simulink model "pd_discreto"  (R2025b)
settings: Solver=VariableStepAuto  StartTime=0.0  StopTime=3  RelTol=1e-3
libraries: simulink x4
settings Model: Creator=rel  LastModifiedBy=rel

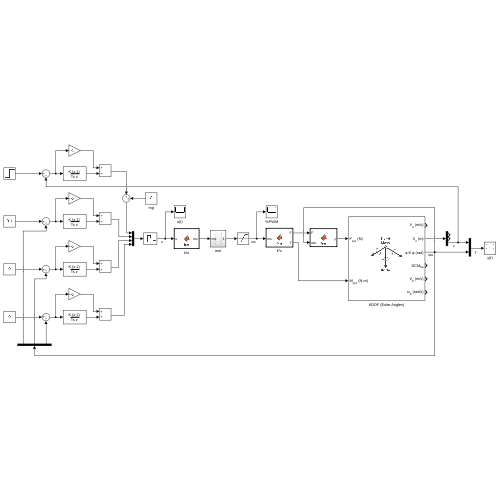
[thumbnail: Simulink's stored preview of the top-level diagram]
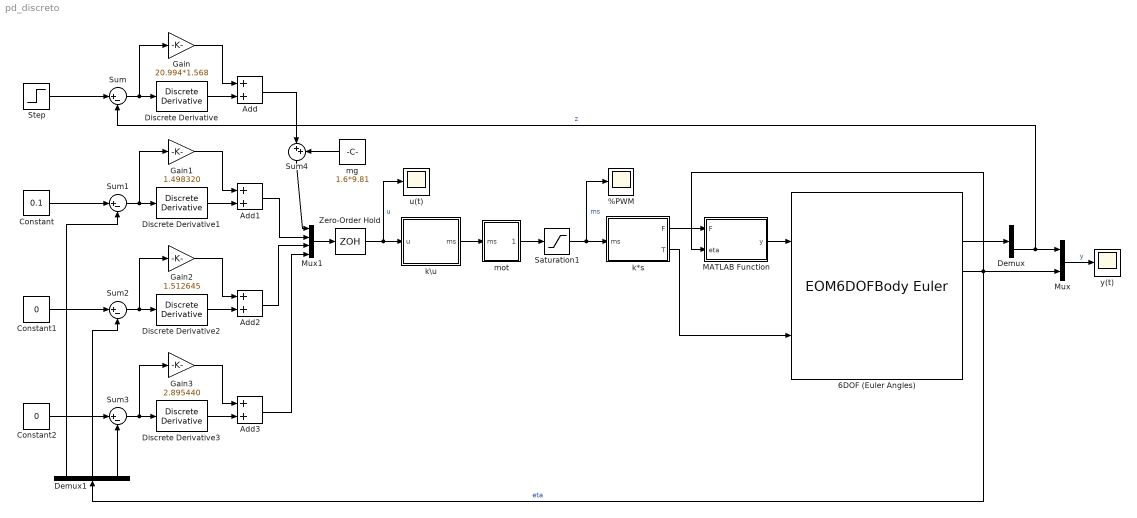
== system pd_discreto ==
  %PWM : Scope
      settings: ActiveDisplayYMinimum=-1  ActiveDisplayYMaximum=1  DataLoggingVariableName=ScopeData4
  6DOF (Euler Angles) : EOM6DOFBodyEuler  mass_0=1.6  inertia=diag([0.021915027 0.022124548 0.042349865])
  Add{,1..3} (4 alike) : Sum
  Constant : Constant  Value=0.1
  Constant1 : Constant  Value=0
  Constant2 : Constant  Value=0
  Demux : Demux  Outputs=3
  Demux1 : Demux  Outputs=3
  Discrete Derivative : simulink/Discrete/Discrete Derivative  gainval=20.994  ICPrevScaledInput=0.0  OutMin=[]  OutMax=[]  OutDataType=fixdt(1, 16)  OutScaling=2^-10  DoSatur=off
  Discrete Derivative1 : simulink/Discrete/Discrete Derivative  gainval=0.352480  ICPrevScaledInput=0.0  OutMin=[]  OutMax=[]  OutDataType=fixdt(1, 16)  OutScaling=2^-10  DoSatur=off
  Discrete Derivative2 : simulink/Discrete/Discrete Derivative  gainval=0.355850  ICPrevScaledInput=0.0  OutMin=[]  OutMax=[]  OutDataType=fixdt(1, 16)  OutScaling=2^-10  DoSatur=off
  Discrete Derivative3 : simulink/Discrete/Discrete Derivative  gainval=0.681153  ICPrevScaledInput=0.0  OutMin=[]  OutMax=[]  OutDataType=fixdt(1, 16)  OutScaling=2^-10  DoSatur=off
  Gain : Gain  Gain=20.994*1.568
  Gain1 : Gain  Gain=1.498320
  Gain2 : Gain  Gain=1.512645
  Gain3 : Gain  Gain=2.895440
  MATLAB Function : MATLAB Function  TreatAsAtomicUnit=on
  Mux : Mux  Inputs=2
  Mux1 : Mux
  Saturation1 : Saturate  UpperLimit=1  LowerLimit=0
  Step : Step  SampleTime=0
  Sum{,1..3} (4 alike) : Sum  Inputs=|+-
  Sum4 : Sum  Inputs=|++
  Zero-Order Hold : ZeroOrderHold  SampleTime=1/250
  k*s : MATLAB Function  TreatAsAtomicUnit=on
  k\u : MATLAB Function  TreatAsAtomicUnit=on
  mg : Constant  Value=1.6*9.81
  mot : Subsystem
  u(t) : Scope
      settings: ActiveDisplayYMinimum=-11.443750265747013  ActiveDisplayYMaximum=40.270145370877117
  y(t) : Scope
      settings: ActiveDisplayYMinimum=-0.13581717833379781  ActiveDisplayYMaximum=1.0804081084613255
  wires:
  6DOF (Euler Angles)/2 -> Demux/1
  6DOF (Euler Angles)/3 -> MATLAB Function/2(eta), Mux/2, Demux1/1  "eta"
  mot/1(Out1) -> Saturation1/1
  k\u/1(ms) -> mot/1(ms)
  Saturation1/1 -> %PWM/1, k*s/1(ms)  "ms"
  k*s/2(T) -> 6DOF (Euler Angles)/2
  k*s/1(F) -> MATLAB Function/1(F)
  MATLAB Function/1(y) -> 6DOF (Euler Angles)/1
  Sum/1 -> Gain/1, Discrete Derivative/1
  Discrete Derivative/1 -> Add/2
  Gain/1 -> Add/1
  Mux1/1 -> Zero-Order Hold/1
  Zero-Order Hold/1 -> u(t)/1, k\u/1(u)  "u"
  Discrete Derivative1/1 -> Add1/2
  Sum1/1 -> Gain1/1, Discrete Derivative1/1
  Gain1/1 -> Add1/1
  Discrete Derivative2/1 -> Add2/2
  Sum2/1 -> Gain2/1, Discrete Derivative2/1
  Gain2/1 -> Add2/1
  Discrete Derivative3/1 -> Add3/2
  Sum3/1 -> Gain3/1, Discrete Derivative3/1
  Gain3/1 -> Add3/1
  Demux1/1 -> Sum1/2
  Demux1/2 -> Sum2/2
  Demux1/3 -> Sum3/2
  Add1/1 -> Mux1/2
  Add2/1 -> Mux1/3
  Add3/1 -> Mux1/4
  Demux/3 -> Sum/2, Mux/1  "z"
  Mux/1 -> y(t)/1  "y"
  Step/1 -> Sum/1
  Constant1/1 -> Sum2/1
  Constant2/1 -> Sum3/1
  Constant/1 -> Sum1/1
  Add/1 -> Sum4/1
  Sum4/1 -> Mux1/1
  mg/1 -> Sum4/2

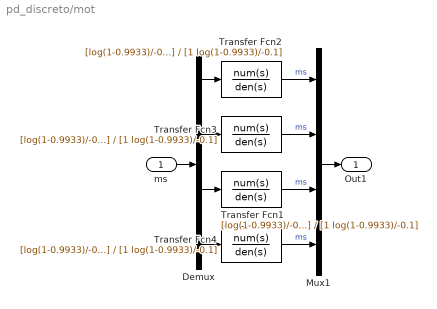
== system pd_discreto/mot ==
  ms : Inport
  Demux : Demux
  Mux1 : Mux
  Transfer Fcn{1..4} (4 alike) : TransferFcn  Numerator=[log(1-0.9933)/-0.1]  Denominator=[1 log(1-0.9933)/-0.1]
  Out1 : Outport
  wires:
  Transfer Fcn3/1 -> Mux1/2  "ms"
  Transfer Fcn1/1 -> Mux1/3  "ms"
  Demux/3 -> Transfer Fcn1/1
  Transfer Fcn4/1 -> Mux1/4  "ms"
  Demux/4 -> Transfer Fcn4/1
  Mux1/1 -> Out1/1
  Transfer Fcn2/1 -> Mux1/1  "ms"
  Demux/2 -> Transfer Fcn3/1
  Demux/1 -> Transfer Fcn2/1
  ms/1 -> Demux/1

== matlab function pd_discreto/k\u ==
  data: u input; ms output
function ms = fcn(u)
% L = 0.0080;
% kF = 0.1600*9.81;
% kM = 0.0086;
L = 0.268554;
kF = 0.7*9.81;
kM = 0.2;
A = [kF kF kF kF; -L*kF -L*kF L*kF L*kF; L*kF -L*kF -L*kF L*kF; -kM kM -kM kM];
ms = A\[u(1); u(2:end)];

== matlab function pd_discreto/MATLAB Function ==
  data: F input; y output; eta input
function y = fcn(F, eta)
phi = eta(1);
theta = eta(2);
psi = eta(3);
y = [0;0;-1.6*9.81] + [sin(theta)*cos(psi) + sin(phi)*cos(theta)*sin(psi); ...
                    sin(theta)*sin(psi) - sin(phi)*cos(theta)*cos(psi); ...
                    cos(phi)*cos(theta)]*F;

== matlab function pd_discreto/k*s ==
  data: ms input; F output; T output
function [F, T] = fcn(ms)
% L = 0.0080;
% kF = 0.1600*9.81;
% kM = 0.0086;
L = 0.268554;
kF = 0.7*9.81;
kM = 0.2;
A = [kF kF kF kF; -L*kF -L*kF L*kF L*kF; L*kF -L*kF -L*kF L*kF; -kM kM -kM kM];
y = A*ms;
F = y(1);
T = y(2:end);
